simulink model "untitled"  (R2019a)
settings: Solver=ode45  StartTime=0.0  StopTime=100  MaxStep=0.2  RelTol=1e-3
settings Model: Creator=mecof  LastModifiedBy=mecof

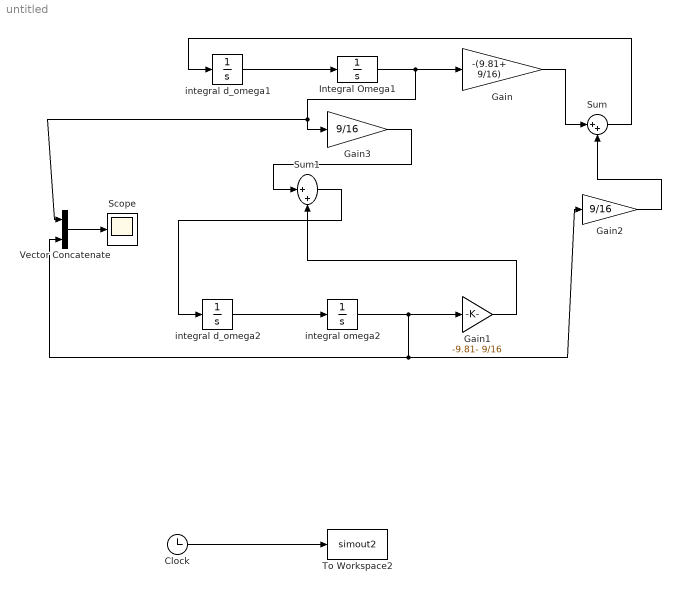
== system untitled ==
  Clock : Clock
  Gain : Gain  Gain=-(9.81+ 9/16)
  Gain1 : Gain  Gain=-9.81- 9/16
  Gain2 : Gain  Gain=9/16
  Gain3 : Gain  Gain=9/16
  Integral Omega1 : Integrator  InitialCondition=[5]  ContinuousStateAttributes=d_theta
  Scope : Scope
  Sum : Sum  Inputs=|++
  Sum1 : Sum  Inputs=|++
  To Workspace2 : ToWorkspace  VariableName=simout2  SaveFormat=Timeseries  SampleTime=-1
  Vector Concatenate : Concatenate
  integral d_omega1 : Integrator  InitialCondition=[0]
  integral d_omega2 : Integrator
  integral omega2 : Integrator
  wires:
  integral d_omega1/1 -> Integral Omega1/1
  Integral Omega1/1 -> Vector Concatenate/1, Gain3/1, Gain/1
  integral omega2/1 -> Vector Concatenate/2, Gain2/1, Gain1/1
  integral d_omega2/1 -> integral omega2/1
  Gain/1 -> Sum/1
  Gain2/1 -> Sum/2
  Sum/1 -> integral d_omega1/1
  Gain1/1 -> Sum1/2
  Sum1/1 -> integral d_omega2/1
  Gain3/1 -> Sum1/1
  Clock/1 -> To Workspace2/1
  Vector Concatenate/1 -> Scope/1
